simulink model "dc"  (R2023b)
settings: Solver=FixedStepAuto  StartTime=0.0  StopTime=10.0  FixedStep=Ts  RelTol=1e-3
values from neighbouring files (symbols this model uses):
  J = 0.02    [dcmotor_control.m]
  Kb = 0.1    [dcmotor_control.m]
  Kf = 0.2    [dcmotor_control.m]
  Km = 0.1    [dcmotor_control.m]
  Kp = 100    [dcmotor_control.m]
  L = 0.5    [dcmotor_control.m]
  R = 2.0    (= 2)    [dcmotor_control.m]
  Vlim = 12    [dcmotor_control.m]
undefined symbols (not defined in the file or in its folder): KI
settings Model: Creator=yeoseojeong  LastModifiedBy=yeoseojeong

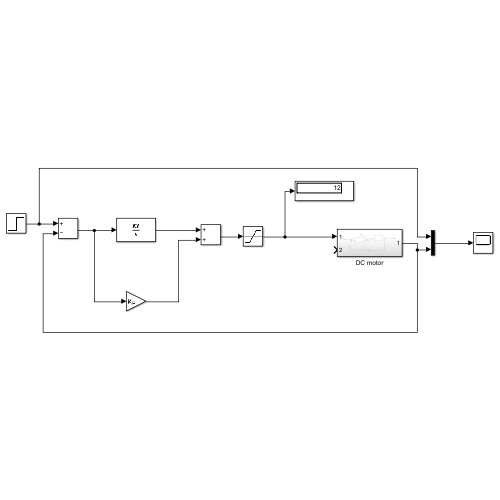
[thumbnail: Simulink's stored preview of the top-level diagram]
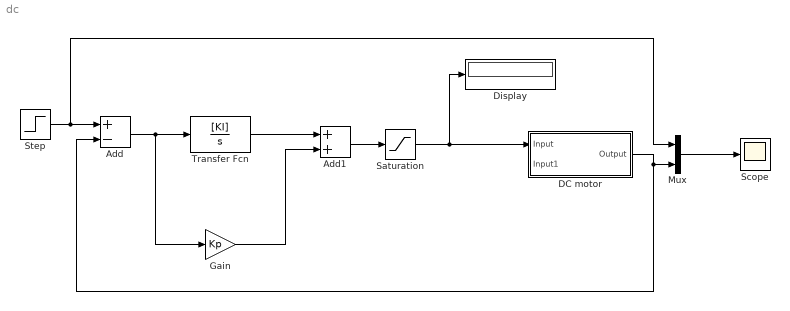
== system dc ==
  Add : Sum  Inputs=+-
  Add1 : Sum
  DC motor : Subsystem
  Display : Display
  Gain : Gain  Gain=Kp
  Mux : Mux  Inputs=2
  Saturation : Saturate  UpperLimit=Vlim  LowerLimit=0
  Scope : Scope
  Step : Step  After=100  SampleTime=0
  Transfer Fcn : TransferFcn  Numerator=[KI]  Denominator=[1 0]
  wires:
  Step/1 -> Mux/1, Add/1
  Add/1 -> Gain/1, Transfer Fcn/1
  Transfer Fcn/1 -> Add1/1
  Mux/1 -> Scope/1
  Gain/1 -> Add1/2
  Add1/1 -> Saturation/1
  Saturation/1 -> Display/1, DC motor/1(Input)
  DC motor/1(Output) -> Mux/2, Add/2

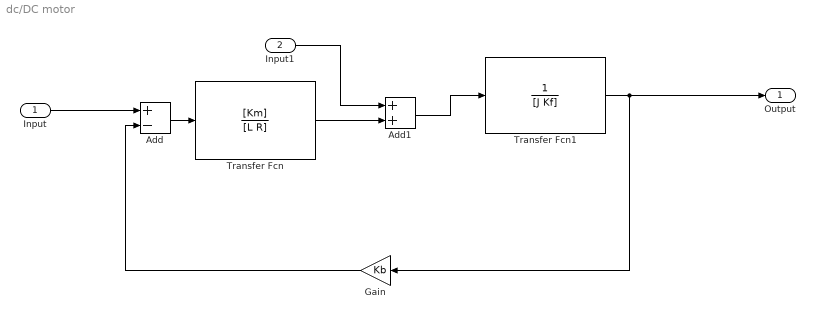
== system dc/DC motor ==
  Input : Inport
  Input1 : Inport  Port=2
  Add : Sum  Inputs=+-
  Add1 : Sum
  Gain : Gain  Gain=Kb
  Transfer Fcn : TransferFcn  Numerator=[Km]  Denominator=[L R]
  Transfer Fcn1 : TransferFcn  Denominator=[J Kf]
  Output : Outport
  wires:
  Add/1 -> Transfer Fcn/1
  Input1/1 -> Add1/1
  Input/1 -> Add/1
  Transfer Fcn/1 -> Add1/2
  Add1/1 -> Transfer Fcn1/1
  Gain/1 -> Add/2
  Transfer Fcn1/1 -> Gain/1, Output/1
